simulink model "Guiagem_Cessna_2024_Hinf_MC_2.sil1-89925"  (R2020b)
settings: Solver=FixedStepAuto  StartTime=0.0  StopTime=100  RelTol=1e-3  EnableMultiTasking=on
undefined symbols (not defined in the file): f, K, Kext
libraries: slrealtimeutilitieslib x4, dspnetwork x1, instrumentlib x1, dspswit3 x1
settings Model: Creator=Sergio  LastModifiedBy=amarc
settings SolverCC: ZeroCrossAlgorithm=Non-adaptive  AutoInsertRateTranBlk=on
settings DataIOCC: SaveFormat=Array  SignalLoggingSaveFormat=ModelDataLogs  ReturnWorkspaceOutputs=off
settings OptimizationCC: ExpressionDepthLimit=2147483647  InitFltsAndDblsToZero=on  LifeSpan=inf
settings DebuggingCC: UnderspecifiedInitializationDetection=Classic  MergeDetectMultiDrivingBlocksExec=none  SolverPrmCheckMsg=warning  FcnCallInpInsideContextMsg=warning  StateNameClashWarn=warning  SFUnexpectedBacktrackingDiag=warning  SFNoUnconditionalDefaultTransitionDiag=warning  SFExecutionAtInitializationDiag=none  ArithmeticOperatorsInVariantConditions=warning
settings HardwareCC: ProdBitPerPointer=32  ProdBitPerSizeT=32  ProdBitPerPtrDiffT=32  ProdLargestAtomicFloat=None  ProdIntDivRoundTo=Undefined  ProdEndianess=Unspecified  ProdWordSize=32  ProdHWDeviceType=32-bit Generic
settings ModelReferenceCC: PropagateSignalLabelsOutOfModel=off
settings CodeAppCC: StateflowObjectComments=on
settings GRTTargetCC: TargetLangStandard=C89/C90 (ANSI)  CombineOutputUpdateFcns=off  GRTInterface=on
settings ConfigComp: CovMetricSettings=dw  CovSaveCumulativeToWorkspaceVar=on  CovSaveSingleToWorkspaceVar=on

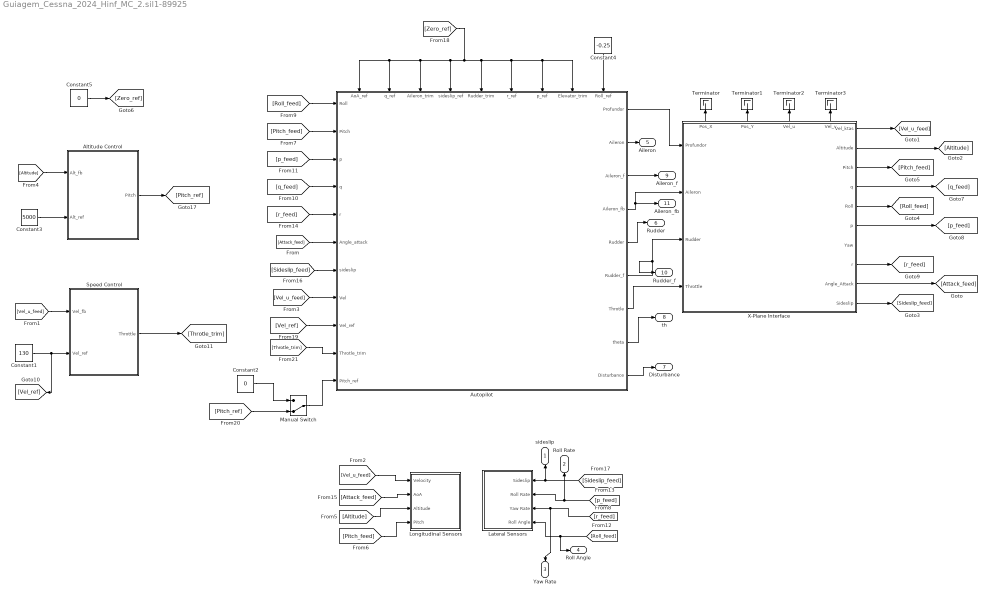
== system Guiagem_Cessna_2024_Hinf_MC_2.sil1-89925 ==
  " X-Plane Interface" : Subsystem
      settings: PortSchema="{\"entries\":[{\"content\":{\"sides\":[{\"content\":{\"connectorIds\":[\"Out11\",\"Out12\",\"Out13\",\"Out14\"]},\"type\":\"ConnectorPlacement.EquallySpacedRectSide\",\"uuid\":\"b287e413-66a9-459c-a605-f8faf73f9bc2\"},{\"content\":{\"connectorIds\":[],\"side\":\"RIGHT\"},\"type\":\"ConnectorPlacement.EquallySpacedRectSide\",\"uuid\":\"a5e9f4a4-94bd-4eea-a928-8343143dc0b5\"},{\"content\":{\"connectorIds\":[\"In1\",\"In2\",\"In3\",\"In4\"],\"side\":\"TOP\"},\"type\":\"ConnectorPlacement.EquallySpacedRectSide\",\"uuid\":\"65fac83d-8715-4b62-9066-f37b198650c3\"},{\"content\":{\"connectorIds\":[\"Out1\",\"Out2\",\"Out3\",\"Out4\",\"Out5\",\"Out6\",\"Out7\",\"Out8\",\"Out9\",\"Out10\"],\"side\":\"BOTTOM\"},\"type\":\"ConnectorPlacement.EquallySpacedRectSide\",\"uuid\":\"a2dcd193-bd07-4351-bec8-c331219c4654\"},{\"content\":{\"connectorIds\":[],\"side\":\"HIDDEN\"},\"type\":\"ConnectorPlacement.EquallySpacedRectSide\",\"uuid\":\"1a5040b2-fe36-41dc-86fb-013b5c75b469\"}]},\"type\":\"ConnectorPlacement.EquallySpacedConnector\",\"uuid\":\"106c77f0-a37d-45d1-adde-f758d3a1985d\"}],\"packageUris\":[\"http://schema.mathworks.com/mf0/Connector/R2020b\"],\"version\":\"1.0\"}"
  Altitude Control : Subsystem
  Autopilot : Subsystem
      settings: PortSchema="{\"entries\":[{\"content\":{\"sides\":[{\"content\":{\"connectorIds\":[\"In1\",\"In2\",\"In3\",\"In4\",\"In5\",\"In6\",\"In7\",\"In8\",\"In9\"]},\"type\":\"ConnectorPlacement.EquallySpacedRectSide\",\"uuid\":\"90d188e5-ac80-4fa1-9be5-1977b7afda35\"},{\"content\":{\"connectorIds\":[],\"side\":\"RIGHT\"},\"type\":\"ConnectorPlacement.EquallySpacedRectSide\",\"uuid\":\"3c236712-b96b-412a-bd89-43ab7dbf8775\"},{\"content\":{\"connectorIds\":[\"In10\",\"In11\",\"In12\",\"In13\",\"In14\",\"In15\",\"In16\",\"In17\",\"In18\",\"In19\",\"In20\"],\"side\":\"TOP\"},\"type\":\"ConnectorPlacement.EquallySpacedRectSide\",\"uuid\":\"6007b185-c294-4b33-95b4-cce134aab69e\"},{\"content\":{\"connectorIds\":[\"Out1\",\"Out2\",\"Out3\",\"Out4\",\"Out5\",\"Out6\",\"Out7\",\"Out8\",\"Out9\"],\"side\":\"BOTTOM\"},\"type\":\"ConnectorPlacement.EquallySpacedRectSide\",\"uuid\":\"8021ee20-ed9f-44e6-9633-5f26e44b493a\"},{\"content\":{\"connectorIds\":[],\"side\":\"HIDDEN\"},\"type\":\"ConnectorPlacement.EquallySpacedRectSide\",\"uuid\":\"d76e2603-a0b8-4e8e-9a67-23be50d7a88d\"}]},\"type\":\"ConnectorPlacement.EquallySpacedConnector\",\"uuid\":\"5cc68935-0bb4-4dc0-b853-f412eb7ddb59\"}],\"packageUris\":[\"http://schema.mathworks.com/mf0/Connector/R2020b\"],\"version\":\"1.0\"}"
  Constant1 : Constant  Value=130
  Constant2 : Constant  Value=0
  Constant3 : Constant  Value=5000
  Constant4 : Constant  Value=-0.25
  Constant5 : Constant  Value=0
  Lateral Sensors : Subsystem
      settings: PortSchema="{\"entries\":[{\"content\":{\"sides\":[{\"content\":{\"connectorIds\":[]},\"type\":\"ConnectorPlacement.EquallySpacedRectSide\",\"uuid\":\"986c3f4b-ed7a-4ad8-bd03-91912b97fe30\"},{\"content\":{\"connectorIds\":[\"In1\",\"In2\",\"In3\",\"In4\"],\"side\":\"RIGHT\"},\"type\":\"ConnectorPlacement.EquallySpacedRectSide\",\"uuid\":\"64bd5685-5cfd-4001-81bc-54a3daf5c9ef\"},{\"content\":{\"connectorIds\":[],\"side\":\"TOP\"},\"type\":\"ConnectorPlacement.EquallySpacedRectSide\",\"uuid\":\"1795adf4-0013-4b9c-8eea-2acf118ad1a4\"},{\"content\":{\"connectorIds\":[],\"side\":\"HIDDEN\"},\"type\":\"ConnectorPlacement.EquallySpacedRectSide\",\"uuid\":\"52ac3bc6-5824-4ddb-b53d-3df0f347e745\"}]},\"type\":\"ConnectorPlacement.EquallySpacedConnector\",\"uuid\":\"dda1921c-f3e4-455c-9a4a-8ad91fc2a8d4\"}],\"packageUris\":[\"http://schema.mathworks.com/mf0/Connector/R2020b\"],\"version\":\"1.0\"}"
  Longitudinal Sensors : Subsystem
  Manual Switch : ManualSwitch  CurrentSetting=0
  Speed Control : Subsystem
  Terminator{,1..3} (4 alike) : Terminator
  sideslip : Outport
  Roll Rate : Outport  Port=2
  Yaw Rate : Outport  Port=3
  Roll Angle : Outport  Port=4
  Aileron : Outport  Port=5
  Rudder : Outport  Port=6
  Disturbance : Outport  Port=7
  th : Outport  Port=8
  Aileron_f : Outport  Port=9
  Rudder_f : Outport  Port=10
  Aileron_fb : Outport  Port=11
  wires:
  Constant1/1 -> Speed Control/1(Vel_ref), [Vel_ref]
  Constant3/1 -> Altitude Control/2(Alt_ref)
  " X-Plane Interface"/9(Angle_Attack) -> [Attack_feed]
  [Attack_feed] -> Autopilot/15(Angle_attack)
  " X-Plane Interface"/1(Vel_ktas) -> [Vel_u_feed]
  [Vel_u_feed] -> Longitudinal Sensors/1(Velocity)
  [Vel_u_feed] -> Autopilot/17(Vel)
  " X-Plane Interface"/2(Altitude) -> [Altitude]
  [Altitude] -> Altitude Control/1(Alt_fb)
  [Altitude] -> Longitudinal Sensors/3(Altitude)
  " X-Plane Interface"/3(Pitch) -> [Pitch_feed]
  [Pitch_feed] -> Longitudinal Sensors/4(Pitch)
  [Pitch_feed] -> Autopilot/11(Pitch)
  " X-Plane Interface"/4(q) -> [q_feed]
  [q_feed] -> Autopilot/13(q)
  " X-Plane Interface"/5(Roll) -> [Roll_feed]
  [Roll_feed] -> Autopilot/10(Roll)
  [Roll_feed] -> Roll Angle/1, Lateral Sensors/4(Roll Angle)
  " X-Plane Interface"/6(p) -> [p_feed]
  [p_feed] -> Autopilot/12(p)
  " X-Plane Interface"/8(r) -> [r_feed]
  [r_feed] -> Autopilot/14(r)
  [Attack_feed] -> Longitudinal Sensors/2(AoA)
  " X-Plane Interface"/10(Sideslip) -> [Sideslip_feed]
  [Sideslip_feed] -> Autopilot/16(sideslip)
  Autopilot/1(Profundor) -> " X-Plane Interface"/1(Profundor)
  Autopilot/4(Aileron_fb) -> " X-Plane Interface"/2(Aileron), Aileron_fb/1
  Autopilot/6(Rudder_f) -> Rudder_f/1, " X-Plane Interface"/3(Rudder)
  Autopilot/7(Throtle) -> " X-Plane Interface"/4(Throttle)
  [Sideslip_feed] -> sideslip/1, Lateral Sensors/1(Sideslip)
  [p_feed] -> Roll Rate/1, Lateral Sensors/2(Roll Rate)
  [r_feed] -> Yaw Rate/1, Lateral Sensors/3(Yaw Rate)
  Manual Switch/1 -> Autopilot/20(Pitch_ref)
  Constant2/1 -> Manual Switch/1
  [Pitch_ref] -> Manual Switch/2
  Altitude Control/1(Pitch) -> [Pitch_ref]
  Constant5/1 -> [Zero_ref]
  [Vel_ref] -> Autopilot/18(Vel_ref)
  [Zero_ref] -> Autopilot/8(Elevator_trim), Autopilot/7(p_ref), Autopilot/6(r_ref), Autopilot/5(Rudder_trim), Autopilot/4(sideslip_ref), Autopilot/3(Aileron_trim), Autopilot/2(q_ref), Autopilot/1(AoA_ref)
  " X-Plane Interface"/11(Pos_X) -> Terminator/1
  " X-Plane Interface"/12(Pos_Y) -> Terminator1/1
  " X-Plane Interface"/13(Vel_u) -> Terminator2/1
  " X-Plane Interface"/14(Vel_v) -> Terminator3/1
  [Throtle_trim] -> Autopilot/19(Throtle_trim)
  Speed Control/1(Throttle) -> [Throtle_trim]
  [Vel_u_feed] -> Speed Control/2(Vel_fb)
  Autopilot/9(Disturbance) -> Disturbance/1
  Autopilot/8(theta) -> th/1
  Constant4/1 -> Autopilot/9(Roll_ref)
  Autopilot/2(Aileron) -> Aileron/1
  Autopilot/5(Rudder) -> Rudder/1
  Autopilot/3(Aileron_f) -> Aileron_f/1

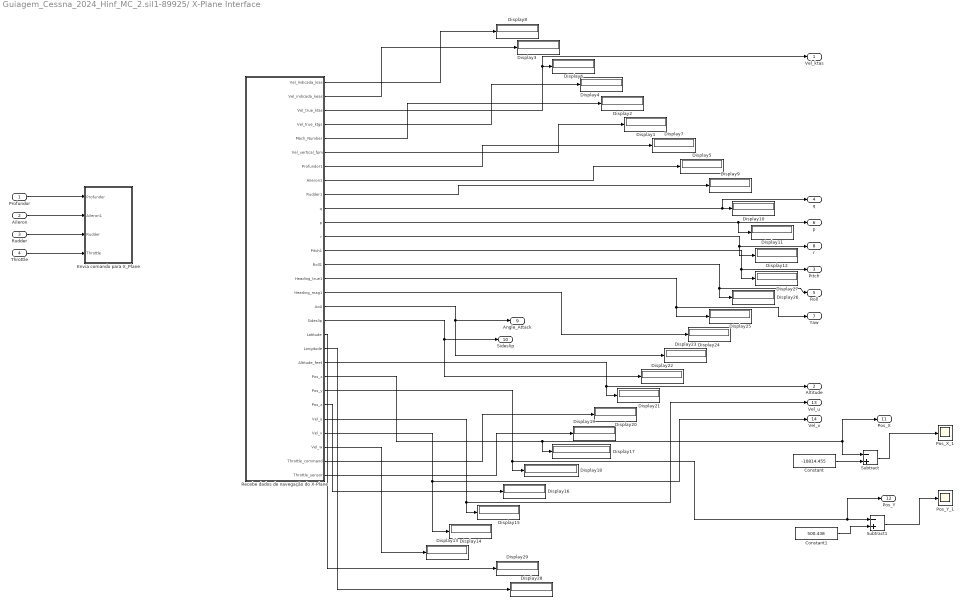
== system Guiagem_Cessna_2024_Hinf_MC_2.sil1-89925/ X-Plane Interface ==
  Profundor : Inport
  Aileron : Inport  Port=2
  Rudder : Inport  Port=3
  Throttle : Inport  Port=4
  Constant : Constant  Value=-10814.455
  Constant1 : Constant  Value=500.438
  Display{1..29} (29 alike) : Display
  Envia comando para X_Plane : Subsystem
  Pos_X_1 : Scope
  Pos_Y_1 : Scope
  Recebe dados de navegação do X-Plane : Subsystem
  Subtract : Sum  Inputs=-+
  Subtract1 : Sum  Inputs=-+
  Vel_ktas : Outport
  Altitude : Outport  Port=2
  Pitch : Outport  Port=3
  q : Outport  Port=4
  Roll : Outport  Port=5
  p : Outport  Port=6
  Yaw : Outport  Port=7
  r : Outport  Port=8
  Angle_Attack : Outport  Port=9
  Sideslip : Outport  Port=10
  Pos_X : Outport  Port=11
  Pos_Y : Outport  Port=12
  Vel_u : Outport  Port=13
  Vel_v : Outport  Port=14
  wires:
  Recebe dados de navegação do X-Plane/13(Pitch1) -> Display27/1, Pitch/1
  Recebe dados de navegação do X-Plane/16(Heading_mag1) -> Display24/1
  Recebe dados de navegação do X-Plane/15(Heading_true1) -> Display25/1, Yaw/1
  Recebe dados de navegação do X-Plane/21(Altitude_feet) -> Display21/1, Altitude/1
  Recebe dados de navegação do X-Plane/12(r) -> Display12/1, r/1
  Recebe dados de navegação do X-Plane/9(Rudder1) -> Display9/1
  Recebe dados de navegação do X-Plane/25(Vel_u) -> Display15/1, Vel_u/1
  Recebe dados de navegação do X-Plane/17(AoA) -> Angle_Attack/1, Display23/1
  Recebe dados de navegação do X-Plane/10(q) -> q/1, Display10/1
  Recebe dados de navegação do X-Plane/22(Pos_x) -> Display17/1, Subtract/1, Pos_X/1
  Recebe dados de navegação do X-Plane/18(Sideslip) -> Sideslip/1, Display22/1
  Recebe dados de navegação do X-Plane/1(Vel_Indicada_kias) -> Display8/1
  Recebe dados de navegação do X-Plane/29(Throttle_sensor) -> Display19/1
  Recebe dados de navegação do X-Plane/24(Pos_z) -> Display16/1
  Recebe dados de navegação do X-Plane/14(Roll1) -> Display26/1, Roll/1
  Recebe dados de navegação do X-Plane/28(Throttle_command) -> Display20/1
  Recebe dados de navegação do X-Plane/27(Vel_w) -> Display13/1
  Recebe dados de navegação do X-Plane/23(Pos_y) -> Display18/1, Pos_Y/1, Subtract1/1
  Recebe dados de navegação do X-Plane/11(p) -> Display11/1, p/1
  Recebe dados de navegação do X-Plane/6(Vel_vertical_fpm) -> Display1/1
  Recebe dados de navegação do X-Plane/2(Vel_indicada_keas) -> Display3/1
  Recebe dados de navegação do X-Plane/8(Aileron1) -> Display5/1
  Recebe dados de navegação do X-Plane/4(Vel_true_ktgs) -> Display4/1
  Recebe dados de navegação do X-Plane/3(Vel_true_ktas) -> Vel_ktas/1, Display6/1
  Recebe dados de navegação do X-Plane/26(Vel_v) -> Display14/1, Vel_v/1
  Recebe dados de navegação do X-Plane/5(Mach_Number) -> Display2/1
  Recebe dados de navegação do X-Plane/7(Profundor1) -> Display7/1
  Subtract/1 -> Pos_X_1/1
  Constant/1 -> Subtract/2
  Constant1/1 -> Subtract1/2
  Subtract1/1 -> Pos_Y_1/1
  Recebe dados de navegação do X-Plane/19(Latitude) -> Display29/1
  Recebe dados de navegação do X-Plane/20(Longitude) -> Display28/1
  Profundor/1 -> Envia comando para X_Plane/1(Profundor)
  Aileron/1 -> Envia comando para X_Plane/2(Aileron1)
  Rudder/1 -> Envia comando para X_Plane/3(Rudder)
  Throttle/1 -> Envia comando para X_Plane/4(Throttle)

== system Guiagem_Cessna_2024_Hinf_MC_2.sil1-89925/Altitude Control ==
  Alt_fb : Inport
  Alt_ref : Inport  Port=2
  Display : Display
  Gain : Gain
  PID Altitude : Subsystem
  Sum2 : Sum  Inputs=|+-  SaturateOnIntegerOverflow=on
  Pitch : Outport
  wires:
  PID Altitude/1(ea) -> Gain/1
  Sum2/1 -> Display/1, PID Altitude/1(e_theta)
  Alt_ref/1 -> Sum2/1
  Alt_fb/1 -> Sum2/2
  Gain/1 -> Pitch/1

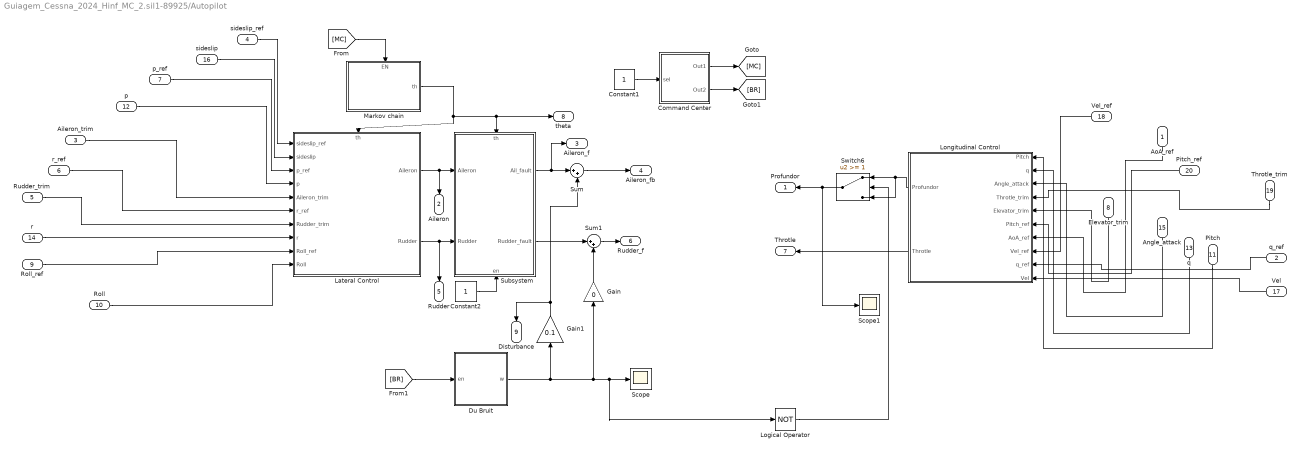
== system Guiagem_Cessna_2024_Hinf_MC_2.sil1-89925/Autopilot ==
  AoA_ref : Inport
  q_ref : Inport  Port=2
  Aileron_trim : Inport  Port=3
  sideslip_ref : Inport  Port=4
  Rudder_trim : Inport  Port=5
  r_ref : Inport  Port=6
  p_ref : Inport  Port=7
  Elevator_trim : Inport  Port=8
  Roll_ref : Inport  Port=9
  Roll : Inport  Port=10
  Pitch : Inport  Port=11
  p : Inport  Port=12
  q : Inport  Port=13
  r : Inport  Port=14
  Angle_attack : Inport  Port=15
  sideslip : Inport  Port=16
  Vel : Inport  Port=17
  Vel_ref : Inport  Port=18
  Throtle_trim : Inport  Port=19
  Pitch_ref : Inport  Port=20
  Command Center : Subsystem
  Constant1 : Constant
  Constant2 : Constant
  Du Bruit : Subsystem
  Gain : Gain  Gain=0
  Gain1 : Gain  Gain=0.1
  Lateral Control : Subsystem
      settings: PortSchema="{\"entries\":[{\"content\":{\"sides\":[{\"content\":{\"connectorIds\":[\"In1\",\"In2\",\"In3\",\"In4\",\"In5\",\"In6\",\"In7\",\"In8\",\"In9\",\"In10\"]},\"type\":\"ConnectorPlacement.EquallySpacedRectSide\",\"uuid\":\"81480b8d-acf9-4486-b64d-17d5a3a359c2\"},{\"content\":{\"connectorIds\":[\"Out1\",\"Out2\"],\"side\":\"RIGHT\"},\"type\":\"ConnectorPlacement.EquallySpacedRectSide\",\"uuid\":\"f51d7c70-ae43-4c04-b132-323ecb9750c2\"},{\"content\":{\"connectorIds\":[\"In11\"],\"side\":\"TOP\"},\"type\":\"ConnectorPlacement.EquallySpacedRectSide\",\"uuid\":\"e45e99c5-9997-4ec4-be29-da73ef44331d\"},{\"content\":{\"connectorIds\":[],\"side\":\"HIDDEN\"},\"type\":\"ConnectorPlacement.EquallySpacedRectSide\",\"uuid\":\"472f75da-d9b5-4c89-82f1-bd7b45161ec6\"}]},\"type\":\"ConnectorPlacement.EquallySpacedConnector\",\"uuid\":\"4f90d613-2ea4-447f-9646-109b9180330b\"}],\"packageUris\":[\"http://schema.mathworks.com/mf0/Connector/R2020b\"],\"version\":\"1.0\"}"
  Logical Operator : Logic  Operator=NOT  AllPortsSameDT=off  OutDataTypeStr=boolean
  Longitudinal Control : Subsystem
  Markov chain : Subsystem
      settings: PortSchema="{\"entries\":[{\"content\":{\"sides\":[{\"content\":{\"connectorIds\":[]},\"type\":\"ConnectorPlacement.EquallySpacedRectSide\",\"uuid\":\"80710c7a-07e6-43ae-a398-972a0eb5af13\"},{\"content\":{\"connectorIds\":[\"Out1\"],\"side\":\"RIGHT\"},\"type\":\"ConnectorPlacement.EquallySpacedRectSide\",\"uuid\":\"28b5b092-7e5d-428e-90bd-fdf9ff161332\"},{\"content\":{\"connectorIds\":[\"In1\"],\"side\":\"TOP\"},\"type\":\"ConnectorPlacement.EquallySpacedRectSide\",\"uuid\":\"22863cb7-627c-45e7-8d90-71727f39a809\"},{\"content\":{\"connectorIds\":[],\"side\":\"HIDDEN\"},\"type\":\"ConnectorPlacement.EquallySpacedRectSide\",\"uuid\":\"e7671043-5e22-4c27-8279-fe6d843a7844\"}]},\"type\":\"ConnectorPlacement.EquallySpacedConnector\",\"uuid\":\"bc28ef5d-b311-4d28-80fd-097e2dffd910\"}],\"packageUris\":[\"http://schema.mathworks.com/mf0/Connector/R2020b\"],\"version\":\"1.0\"}"
  Scope : Scope
  Scope1 : Scope
  Subsystem : Subsystem
      settings: PortSchema="{\"entries\":[{\"content\":{\"sides\":[{\"content\":{\"connectorIds\":[\"In1\",\"In2\"]},\"type\":\"ConnectorPlacement.EquallySpacedRectSide\",\"uuid\":\"51a358d2-0277-4e02-9bc5-d86ec75e586a\"},{\"content\":{\"connectorIds\":[\"Out1\",\"Out2\"],\"side\":\"RIGHT\"},\"type\":\"ConnectorPlacement.EquallySpacedRectSide\",\"uuid\":\"48fac5f6-d3f7-4a23-9035-dace107cd9ad\"},{\"content\":{\"connectorIds\":[\"In3\"],\"side\":\"TOP\"},\"type\":\"ConnectorPlacement.EquallySpacedRectSide\",\"uuid\":\"fe2b725a-5173-4175-81cd-54f0c8666ca6\"},{\"content\":{\"connectorIds\":[\"In4\"],\"side\":\"BOTTOM\"},\"type\":\"ConnectorPlacement.EquallySpacedRectSide\",\"uuid\":\"7335eb3f-eaf6-4179-b795-6b8ea5857190\"},{\"content\":{\"connectorIds\":[],\"side\":\"HIDDEN\"},\"type\":\"ConnectorPlacement.EquallySpacedRectSide\",\"uuid\":\"2585f13a-08e3-4863-882a-f65ebe29ac28\"}]},\"type\":\"ConnectorPlacement.EquallySpacedConnector\",\"uuid\":\"792a0ec4-d064-45f9-9106-30d8e1278945\"}],\"packageUris\":[\"http://schema.mathworks.com/mf0/Connector/R2020b\"],\"version\":\"1.0\"}"
  Sum : Sum  Inputs=|++
  Sum1 : Sum  Inputs=|++
  Switch6 : Switch  Threshold=1
  Profundor : Outport
  Aileron : Outport  Port=2
  Aileron_f : Outport  Port=3
  Aileron_fb : Outport  Port=4
  Rudder : Outport  Port=5
  Rudder_f : Outport  Port=6
  Throtle : Outport  Port=7
  theta : Outport  Port=8
  Disturbance : Outport  Port=9
  wires:
  Pitch/1 -> Longitudinal Control/1(Pitch)
  q/1 -> Longitudinal Control/2(q)
  Angle_attack/1 -> Longitudinal Control/3(Angle_attack)
  Throtle_trim/1 -> Longitudinal Control/4(Throtle_trim)
  Elevator_trim/1 -> Longitudinal Control/5(Elevator_trim)
  Pitch_ref/1 -> Longitudinal Control/6(Pitch_ref)
  AoA_ref/1 -> Longitudinal Control/7(AoA_ref)
  Vel_ref/1 -> Longitudinal Control/8(Vel_ref)
  q_ref/1 -> Longitudinal Control/9(q_ref)
  Vel/1 -> Longitudinal Control/10(Vel)
  sideslip_ref/1 -> Lateral Control/1(sideslip_ref)
  sideslip/1 -> Lateral Control/2(sideslip)
  p_ref/1 -> Lateral Control/3(p_ref)
  p/1 -> Lateral Control/4(p)
  Aileron_trim/1 -> Lateral Control/5(Aileron_trim)
  r_ref/1 -> Lateral Control/6(r_ref)
  Rudder_trim/1 -> Lateral Control/7(Rudder_trim)
  r/1 -> Lateral Control/8(r)
  Roll_ref/1 -> Lateral Control/9(Roll_ref)
  Roll/1 -> Lateral Control/10(Roll)
  Lateral Control/1(Aileron) -> Subsystem/1(Aileron), Aileron/1
  Longitudinal Control/2(Throtle) -> Throtle/1
  Lateral Control/2(Rudder) -> Rudder/1, Subsystem/2(Rudder)
  Subsystem/1(Ail_fault) -> Aileron_f/1, Sum/1
  Sum/1 -> Aileron_fb/1
  Subsystem/2(Rudder_fault) -> Sum1/1
  Gain/1 -> Sum1/2
  [MC] -> Markov chain/1(EN)
  Markov chain/1(th) -> theta/1, Subsystem/3(th), Lateral Control/11(th)
  Constant1/1 -> Command Center/1(sel)
  Command Center/2(Out2) -> [BR]
  Command Center/1(Out1) -> [MC]
  Gain1/1 -> Sum/2, Disturbance/1
  [BR] -> Du Bruit/1(en)
  Constant2/1 -> Subsystem/4(en)
  Sum1/1 -> Rudder_f/1
  Switch6/1 -> Scope1/1, Profundor/1
  Longitudinal Control/1(Profundor) -> Switch6/3, Switch6/1
  Du Bruit/1(w) -> Gain1/1, Gain/1, Logical Operator/1, Scope/1
  Logical Operator/1 -> Switch6/2

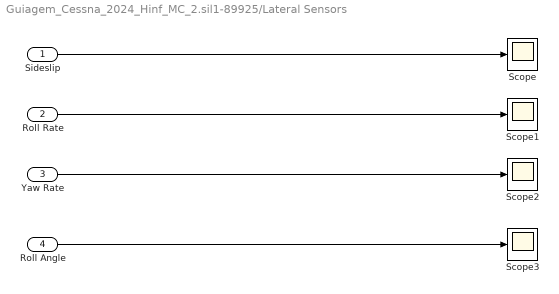
== system Guiagem_Cessna_2024_Hinf_MC_2.sil1-89925/Lateral Sensors ==
  Sideslip : Inport
  Roll Rate : Inport  Port=2
  Yaw Rate : Inport  Port=3
  Roll Angle : Inport  Port=4
  Scope{,1..3} (4 alike) : Scope
  wires:
  Sideslip/1 -> Scope/1
  Roll Rate/1 -> Scope1/1
  Roll Angle/1 -> Scope3/1
  Yaw Rate/1 -> Scope2/1

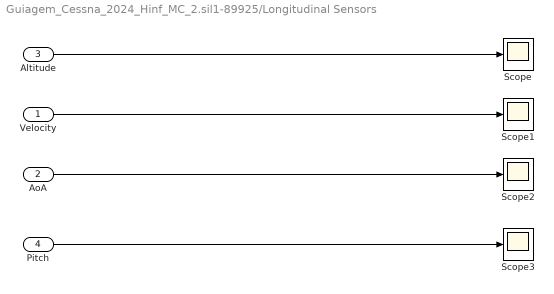
== system Guiagem_Cessna_2024_Hinf_MC_2.sil1-89925/Longitudinal Sensors ==
  Velocity : Inport
  AoA : Inport  Port=2
  Altitude : Inport  Port=3
  Pitch : Inport  Port=4
  Scope{,1..3} (4 alike) : Scope
  wires:
  Altitude/1 -> Scope/1
  Velocity/1 -> Scope1/1
  AoA/1 -> Scope2/1
  Pitch/1 -> Scope3/1

== system Guiagem_Cessna_2024_Hinf_MC_2.sil1-89925/Speed Control ==
  Vel_ref : Inport
  Vel_fb : Inport  Port=2
  PID Velocidade : Subsystem
  Sum7 : Sum  Inputs=|+-
  Throttle : Outport
  wires:
  Vel_fb/1 -> Sum7/2
  PID Velocidade/1(ev) -> Throttle/1
  Vel_ref/1 -> Sum7/1
  Sum7/1 -> PID Velocidade/1(e_vel)

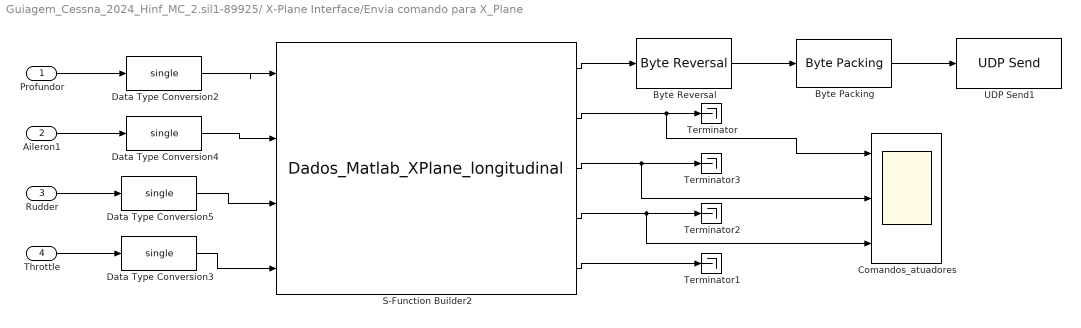
== system Guiagem_Cessna_2024_Hinf_MC_2.sil1-89925/ X-Plane Interface/Envia comando para X_Plane ==
  Profundor : Inport
  Aileron1 : Inport  Port=2
  Rudder : Inport  Port=3
  Throttle : Inport  Port=4
  Byte Packing : slrealtimeutilitieslib/Byte Packing  MaskPackedDataType=uint8  MaskUnpackedDataTypes={'uint8'}  MaskAlignment=1
  Byte Reversal : slrealtimeutilitieslib/Byte Reversal  numInp=1
      settings: SourceProductBaseCode=XP
  Comandos_atuadores : Scope  NumInputPorts=3
  Data Type Conversion{2..5} (4 alike) : DataTypeConversion  OutDataTypeStr=single  SaturateOnIntegerOverflow=on
  S-Function Builder2 : S-Function  InitFcn=try, set_param(gcb,'FunctionName','Dados_Matlab_XPlane_longitudinal'), end  FunctionName=Dados_Matlab_XPlane_longitudinal  SFunctionModules=Dados_Matlab_XPlane_longitudinal_wrapper  SFunctionDeploymentMode=off  EnableBusSupport=off  mask(S-Function Builder){}
      mask help: The S-Function Builder block creates a wrapper C-MEX S-function from your supplied C code with multiple input ports, output ports, and a variable number of scalar, vector, or matrix parameters. The input and output ports can propagate Simulink built-in data types, fixed-point datatypes, complex, frame, 1-D, and 2-D signals. This block also supports discrete and continuous states of type real. You can optionally have the block generate a TLC file to be used with Real-Time Workshop for code generation.
      mask init:
      | val = [[.9  0.75 0.75 1 1 .9 .9 1]',[1 1 0.75 0.75 .9 .9 1 .9]'];try , sys = get_param(gcb,'SfunBuilderFcnName');if isempty(sys), sys = get_param(gcb,'FunctionName'); end,catch, sys = get_param(gcb,'FunctionName'); end
      settings: CopyFcn=set_param(gcbh,'LinkStatus','none')  PreSaveFcn=try, set_param(gcb,'FunctionName','Dados_Matlab_XPlane_longitudinal'), end  OpenFcn=sfunctionwizard(gcbh)
      mask Display: plot(val(:,1),val(:,2)),disp(sys),port_label('input',1,'Profundor'),port_label('input',2,'Aileron'),port_label('input',3,'Rudder'),port_label('input',4,'Throttle'),port_label('output',1,'Atuadores_Out'),port_label('output',2,'elevator_out'),port_label('output',3,'aileron_out'),port_label('output',4,'rudder_out'),port_label('output',5,'throttle_out')
  Terminator{,1..3} (4 alike) : Terminator
  UDP Send1 : dspnetwork/UDP Send  remoteURL='161.24.191.101'  remotePort=49000  localURL='0.0.0.0'  localPortSource=Automatically determine  localPort=-1  sendBufferSize=113  sampletime=-1  blockPlatform=[]  separateLengthPort=0
  wires:
  Data Type Conversion5/1 -> S-Function Builder2/3
  S-Function Builder2/2 -> Terminator/1, Comandos_atuadores/1
  Rudder/1 -> Data Type Conversion5/1
  Aileron1/1 -> Data Type Conversion4/1
  S-Function Builder2/5 -> Terminator1/1
  S-Function Builder2/4 -> Terminator2/1, Comandos_atuadores/3
  S-Function Builder2/3 -> Terminator3/1, Comandos_atuadores/2
  Profundor/1 -> Data Type Conversion2/1
  Byte Reversal/1 -> Byte Packing/1
  Data Type Conversion2/1 -> S-Function Builder2/1
  Data Type Conversion4/1 -> S-Function Builder2/2
  S-Function Builder2/1 -> Byte Reversal/1
  Data Type Conversion3/1 -> S-Function Builder2/4
  Byte Packing/1 -> UDP Send1/1
  Throttle/1 -> Data Type Conversion3/1

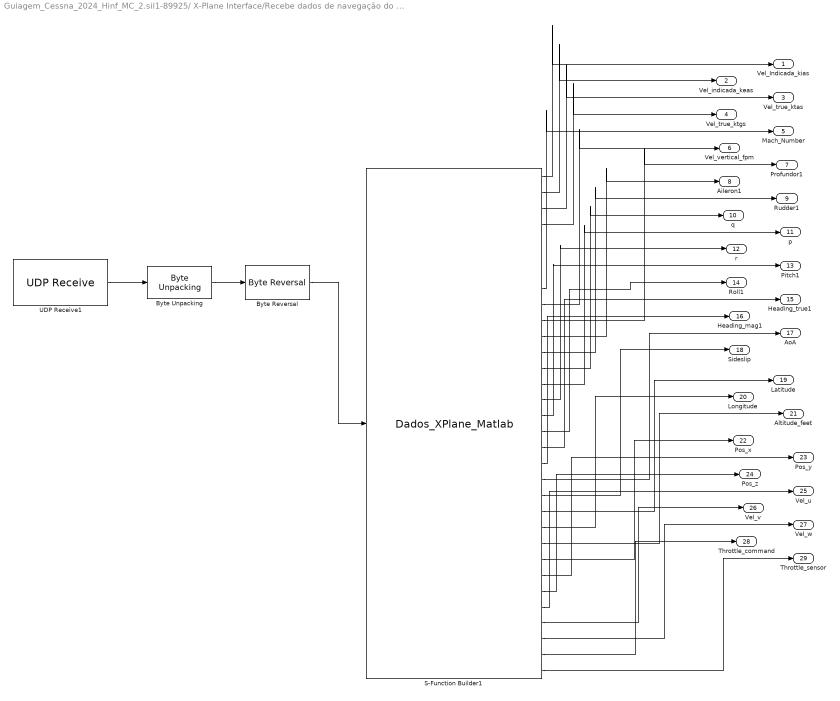
== system Guiagem_Cessna_2024_Hinf_MC_2.sil1-89925/ X-Plane Interface/Recebe dados de navegação do X-Plane ==
  Byte Reversal : slrealtimeutilitieslib/Byte Reversal  numInp=1
      settings: SourceProductBaseCode=XP
  Byte Unpacking : slrealtimeutilitieslib/Byte Unpacking  MaskUnpackedDataTypes={'uint8'}  MaskUnpackedDataSizes={[1, 365]}  MaskAlignment=1
      settings: SourceProductBaseCode=XP
  S-Function Builder1 : S-Function  InitFcn=try, set_param(gcb,'FunctionName','Dados_XPlane_Matlab'), end  FunctionName=Dados_XPlane_Matlab  SFunctionModules=Dados_XPlane_Matlab_wrapper  SFunctionDeploymentMode=off  EnableBusSupport=off  mask(S-Function Builder){}
      mask help: The S-Function Builder block creates a wrapper C-MEX S-function from your supplied C code with multiple input ports, output ports, and a variable number of scalar, vector, or matrix parameters. The input and output ports can propagate Simulink built-in data types, fixed-point datatypes, complex, frame, 1-D, and 2-D signals. This block also supports discrete and continuous states of type real. You can optionally have the block generate a TLC file to be used with Real-Time Workshop for code generation.
      mask init: same as Guiagem_Cessna_2024_Hinf_MC_2.sil1-89925/ X-Plane Interface/Envia comando para X_Plane/S-Function Builder2
      settings: CopyFcn=set_param(gcbh,'LinkStatus','none')  PreSaveFcn=try, set_param(gcb,'FunctionName','Dados_XPlane_Matlab'), end  OpenFcn=sfunctionwizard(gcbh)
      mask Display: plot(val(:,1),val(:,2)),disp(sys),port_label('input',1,'Dados_in'),port_label('output',1,'Vind_kias'),port_label('output',2,'Vind_keas'),port_label('output',3,'Vtrue_ktas'),port_label('output',4,'Vtrue_ktgs'),port_label('output',5,'Vind_mph'),port_label('output',6,'Vtrue_mphas'),port_label('output',7,'Vtrue_mphgs'),port_label('output',8,'Mach'),port_label('output',9,'VVI'),port_label('output',10,'Elevator'),port_label('output',11,'Aileron'),port_label('output',12,'Rudder'),port_label('output',13,'Q'),port_label('output',14,'P'),port_label('output',15,'R'),port_label('output',16,'Pitch'),port_label('output',17,'Roll'),port_label('output',18,'Heading_true'),port_label('output',19,'Heading_mag'),port_label('output',20,'AoA'),port_label('output',21,'Sideslip'),port_label('output',22,'Latitude'),port_label('output',23,'Longitude'),port_label('output',24,'Altitude'),port_label('output',25,'X'),port_label('output',26,'Y'),port_label('output',27,'Z'),port_label('output',28,'Vu'),port_label('output',29,'Vv'),port_label('output',30,'Vw'),port_label('output',31,'Throtle_com'),port_label('output',32,'Throtle_sen')
  UDP Receive1 : instrumentlib/UDP Receive  Host=161.24.191.101  Port=49001  LocalPort=49001  EnablePortSharing=off  GetLatestData=off  DataSize=365  DataType=uint8  ASCIIFormatting=%f,  Terminator=LF  ByteOrder=BigEndian  EnableBlockingMode=on  Timeout=5  SampleTime=0.01  LocalAddress=161.24.191.100
  Vel_Indicada_kias : Outport
  Vel_indicada_keas : Outport  Port=2
  Vel_true_ktas : Outport  Port=3
  Vel_true_ktgs : Outport  Port=4
  Mach_Number : Outport  Port=5
  Vel_vertical_fpm : Outport  Port=6
  Profundor1 : Outport  Port=7
  Aileron1 : Outport  Port=8
  Rudder1 : Outport  Port=9
  q : Outport  Port=10
  p : Outport  Port=11
  r : Outport  Port=12
  Pitch1 : Outport  Port=13
  Roll1 : Outport  Port=14
  Heading_true1 : Outport  Port=15
  Heading_mag1 : Outport  Port=16
  AoA : Outport  Port=17
  Sideslip : Outport  Port=18
  Latitude : Outport  Port=19
  Longitude : Outport  Port=20
  Altitude_feet : Outport  Port=21
  Pos_x : Outport  Port=22
  Pos_y : Outport  Port=23
  Pos_z : Outport  Port=24
  Vel_u : Outport  Port=25
  Vel_v : Outport  Port=26
  Vel_w : Outport  Port=27
  Throttle_command : Outport  Port=28
  Throttle_sensor : Outport  Port=29
  wires:
  Byte Unpacking/1 -> Byte Reversal/1
  Byte Reversal/1 -> S-Function Builder1/1
  UDP Receive1/1 -> Byte Unpacking/1
  S-Function Builder1/1 -> Vel_Indicada_kias/1
  S-Function Builder1/2 -> Vel_indicada_keas/1
  S-Function Builder1/3 -> Vel_true_ktas/1
  S-Function Builder1/4 -> Vel_true_ktgs/1
  S-Function Builder1/10 -> Profundor1/1
  S-Function Builder1/8 -> Mach_Number/1
  S-Function Builder1/9 -> Vel_vertical_fpm/1
  S-Function Builder1/11 -> Aileron1/1
  S-Function Builder1/12 -> Rudder1/1
  S-Function Builder1/13 -> q/1
  S-Function Builder1/14 -> p/1
  S-Function Builder1/15 -> r/1
  S-Function Builder1/16 -> Pitch1/1
  S-Function Builder1/17 -> Roll1/1
  S-Function Builder1/18 -> Heading_true1/1
  S-Function Builder1/19 -> Heading_mag1/1
  S-Function Builder1/20 -> AoA/1
  S-Function Builder1/21 -> Sideslip/1
  S-Function Builder1/22 -> Latitude/1
  S-Function Builder1/23 -> Longitude/1
  S-Function Builder1/24 -> Altitude_feet/1
  S-Function Builder1/25 -> Pos_x/1
  S-Function Builder1/26 -> Pos_y/1
  S-Function Builder1/27 -> Pos_z/1
  S-Function Builder1/28 -> Vel_u/1
  S-Function Builder1/29 -> Vel_v/1
  S-Function Builder1/30 -> Vel_w/1
  S-Function Builder1/31 -> Throttle_command/1
  S-Function Builder1/32 -> Throttle_sensor/1

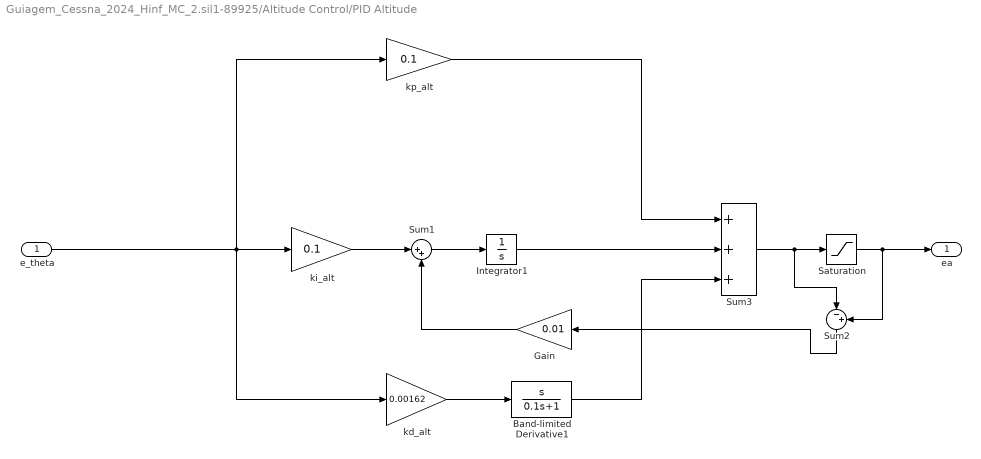
== system Guiagem_Cessna_2024_Hinf_MC_2.sil1-89925/Altitude Control/PID Altitude ==
  e_theta : Inport
  Band-limited Derivative1 : TransferFcn  Numerator=[1 0]  Denominator=[0.1 1]
  Gain : Gain  Gain=0.01
  Integrator1 : Integrator
  Saturation : Saturate  UpperLimit=800  LowerLimit=-800
  Sum1 : Sum  Inputs=|++
  Sum2 : Sum  Inputs=|-+
  Sum3 : Sum  Inputs=+++  InputSameDT=on  SaturateOnIntegerOverflow=on  OutDataTypeStr=Inherit: Same as first input
  kd_alt : Gain  Gain=0.00162  SaturateOnIntegerOverflow=on  OutDataTypeStr=Inherit: Same as input  ParamDataTypeStr=Inherit: Same as input
  ki_alt : Gain  Gain=0.1  SaturateOnIntegerOverflow=on  OutDataTypeStr=Inherit: Same as input  ParamDataTypeStr=Inherit: Same as input
  kp_alt : Gain  Gain=0.1  SaturateOnIntegerOverflow=on  OutDataTypeStr=Inherit: Same as input  ParamDataTypeStr=Inherit: Same as input
  ea : Outport
  wires:
  kp_alt/1 -> Sum3/1
  Band-limited Derivative1/1 -> Sum3/3
  e_theta/1 -> ki_alt/1, kd_alt/1, kp_alt/1
  kd_alt/1 -> Band-limited Derivative1/1
  Integrator1/1 -> Sum3/2
  Sum3/1 -> Sum2/1, Saturation/1
  Saturation/1 -> Sum2/2, ea/1
  ki_alt/1 -> Sum1/1
  Sum1/1 -> Integrator1/1
  Sum2/1 -> Gain/1
  Gain/1 -> Sum1/2

== system Guiagem_Cessna_2024_Hinf_MC_2.sil1-89925/Autopilot/Command Center ==
  sel : Inport
  Demux : Demux  Outputs=2
  MATLAB Function : MATLAB Function  TreatAsAtomicUnit=on
  Out1 : Outport
  Out2 : Outport  Port=2
  wires:
  MATLAB Function/1(y) -> Demux/1
  Demux/1 -> Out1/1
  sel/1 -> MATLAB Function/1(sel)
  Demux/2 -> Out2/1

== system Guiagem_Cessna_2024_Hinf_MC_2.sil1-89925/Autopilot/Du Bruit ==
  en : Inport
  Counter : dspswit3/Counter  Direction=Up  CountEvent=Non-zero sample  CounterSize=User defined  MaxCount=301  InitialCount=0  Output=Count and Hit  HitValue=32  ResetInput=off  SamplesPerFrame=1  Ts=1  CntDtype=double  HitDtype=Logical
  Delay : Delay  DelayLength=1
  MATLAB Function : MATLAB Function  TreatAsAtomicUnit=on
  w : Outport
  wires:
  MATLAB Function/1(w) -> w/1, Delay/1
  Counter/1 -> MATLAB Function/2(cnt)
  Delay/1 -> Counter/1
  en/1 -> MATLAB Function/1(en)

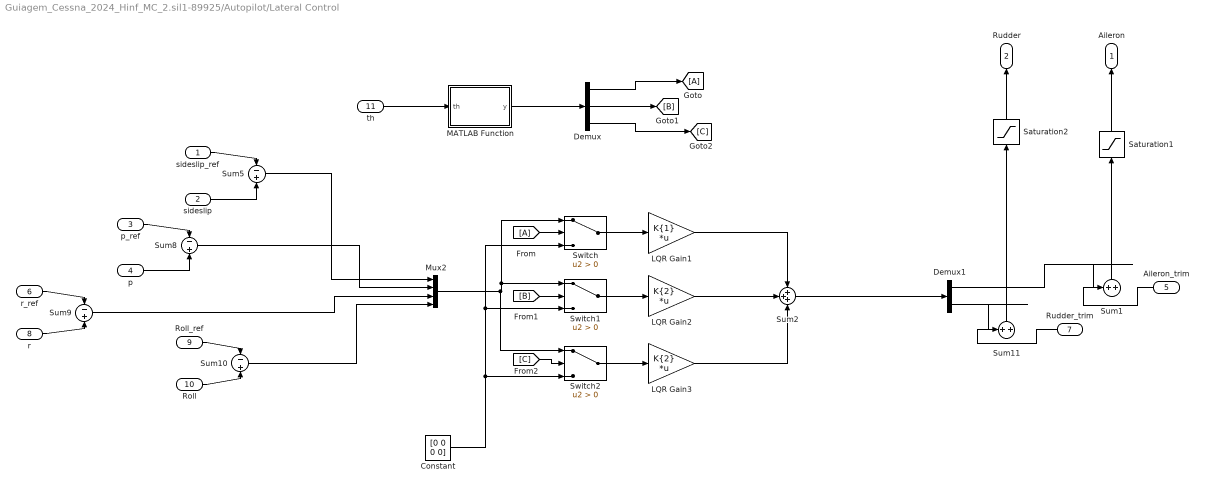
== system Guiagem_Cessna_2024_Hinf_MC_2.sil1-89925/Autopilot/Lateral Control ==
  sideslip_ref : Inport
  sideslip : Inport  Port=2
  p_ref : Inport  Port=3
  p : Inport  Port=4
  Aileron_trim : Inport  Port=5
  r_ref : Inport  Port=6
  Rudder_trim : Inport  Port=7
  r : Inport  Port=8
  Roll_ref : Inport  Port=9
  Roll : Inport  Port=10
  th : Inport  Port=11
  Constant : Constant  Value=[0 0 0 0]  VectorParams1D=off
  Demux : Demux  Outputs=3
  Demux1 : Demux  Outputs=2
  LQR Gain1 : Gain  Gain=K{1}  Multiplication=Matrix(K*u) (u vector)  SaturateOnIntegerOverflow=on  OutDataTypeStr=Inherit: Same as input  ParamDataTypeStr=Inherit: Same as input
  LQR Gain2 : Gain  Gain=K{2}  Multiplication=Matrix(K*u) (u vector)  SaturateOnIntegerOverflow=on  OutDataTypeStr=Inherit: Same as input  ParamDataTypeStr=Inherit: Same as input
  LQR Gain3 : Gain  Gain=K{2}  Multiplication=Matrix(K*u) (u vector)  SaturateOnIntegerOverflow=on  OutDataTypeStr=Inherit: Same as input  ParamDataTypeStr=Inherit: Same as input
  MATLAB Function : MATLAB Function  TreatAsAtomicUnit=on
  Mux2 : Mux
  Saturation1 : Saturate  UpperLimit=1  LowerLimit=-1
  Saturation2 : Saturate  UpperLimit=1  LowerLimit=-1
  Sum1 : Sum  InputSameDT=on  SaturateOnIntegerOverflow=on  OutDataTypeStr=Inherit: Same as first input
  Sum{5,8..10} (4 alike) : Sum  Inputs=-+  InputSameDT=on  SaturateOnIntegerOverflow=on  OutDataTypeStr=Inherit: Same as first input
  Sum11 : Sum  InputSameDT=on  SaturateOnIntegerOverflow=on  OutDataTypeStr=Inherit: Same as first input
  Sum2 : Sum  Inputs=+++  InputSameDT=on  SaturateOnIntegerOverflow=on  OutDataTypeStr=Inherit: Same as first input
  Switch : Switch  Criteria=u2 > Threshold
  Switch1 : Switch  Criteria=u2 > Threshold
  Switch2 : Switch  Criteria=u2 > Threshold
  Aileron : Outport
  Rudder : Outport  Port=2
  wires:
  Demux1/2 -> Sum11/2
  Roll/1 -> Sum10/2
  Sum5/1 -> Mux2/1
  Sum1/1 -> Saturation1/1
  sideslip_ref/1 -> Sum5/1
  Sum11/1 -> Saturation2/1
  sideslip/1 -> Sum5/2
  Saturation1/1 -> Aileron/1
  r/1 -> Sum9/2
  p/1 -> Sum8/2
  Sum9/1 -> Mux2/3
  p_ref/1 -> Sum8/1
  Aileron_trim/1 -> Sum1/1
  Roll_ref/1 -> Sum10/1
  Demux1/1 -> Sum1/2
  Rudder_trim/1 -> Sum11/1
  Saturation2/1 -> Rudder/1
  Sum10/1 -> Mux2/4
  r_ref/1 -> Sum9/1
  Sum8/1 -> Mux2/2
  th/1 -> MATLAB Function/1(th)
  Switch/1 -> LQR Gain1/1
  Switch1/1 -> LQR Gain2/1
  LQR Gain1/1 -> Sum2/1
  LQR Gain2/1 -> Sum2/2
  LQR Gain3/1 -> Sum2/3
  Switch2/1 -> LQR Gain3/1
  Sum2/1 -> Demux1/1
  Mux2/1 -> Switch2/1, Switch1/1, Switch/1
  Constant/1 -> Switch2/3, Switch1/3, Switch/3
  Demux/2 -> [B]
  MATLAB Function/1(y) -> Demux/1
  Demux/3 -> [C]
  Demux/1 -> [A]
  [A] -> Switch/2
  [B] -> Switch1/2
  [C] -> Switch2/2

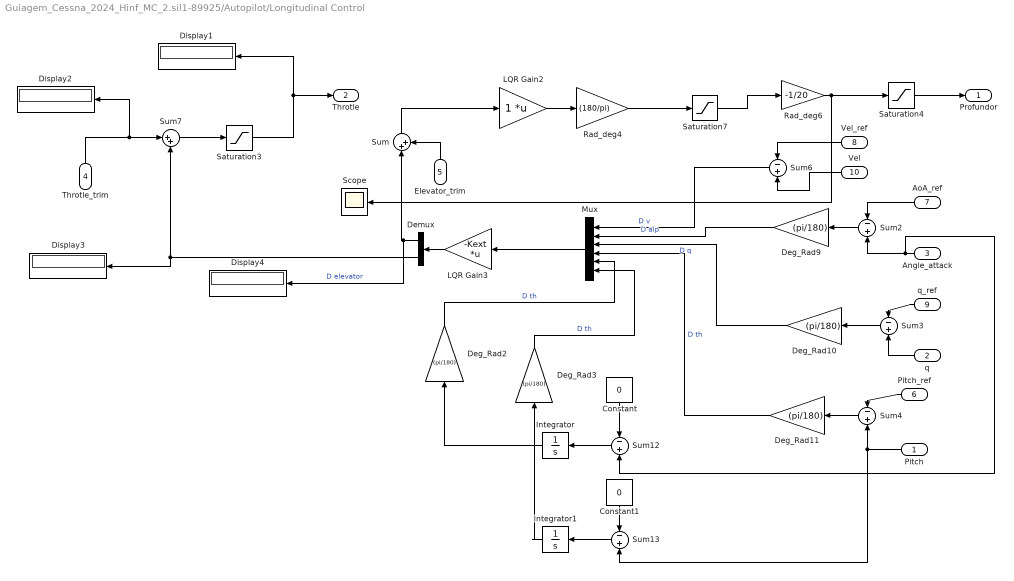
== system Guiagem_Cessna_2024_Hinf_MC_2.sil1-89925/Autopilot/Longitudinal Control ==
  Pitch : Inport
  q : Inport  Port=2
  Angle_attack : Inport  Port=3
  Throtle_trim : Inport  Port=4
  Elevator_trim : Inport  Port=5
  Pitch_ref : Inport  Port=6
  AoA_ref : Inport  Port=7
  Vel_ref : Inport  Port=8
  q_ref : Inport  Port=9
  Vel : Inport  Port=10
  Constant : Constant  Value=0
  Constant1 : Constant  Value=0
  Deg_Rad{2..3,9..11} (5 alike) : Gain  Gain=(pi/180)
  Demux : Demux  Outputs=2
  Display{1..4} (4 alike) : Display
  Integrator : Integrator
  Integrator1 : Integrator
  LQR Gain2 : Gain  Multiplication=Matrix(K*u)  SaturateOnIntegerOverflow=on  OutDataTypeStr=Inherit: Same as input  ParamDataTypeStr=Inherit: Same as input
  LQR Gain3 : Gain  Gain=-Kext  Multiplication=Matrix(K*u)  SaturateOnIntegerOverflow=on  OutDataTypeStr=Inherit: Same as input  ParamDataTypeStr=Inherit: Same as input
  Mux : Mux  Inputs=6
  Rad_deg4 : Gain  Gain=(180/pi)
  Rad_deg6 : Gain  Gain=-1/20
  Saturation3 : Saturate  UpperLimit=1  LowerLimit=0
  Saturation4 : Saturate
  Saturation7 : Saturate  UpperLimit=20  LowerLimit=-20
  Scope : Scope
  Sum : Sum  Inputs=|++
  Sum{2..4,6,12..13} (6 alike) : Sum  Inputs=-+  InputSameDT=on  SaturateOnIntegerOverflow=on  OutDataTypeStr=Inherit: Same as first input
  Sum7 : Sum  Inputs=|++
  Profundor : Outport
  Throtle : Outport  Port=2
  wires:
  Demux/1 -> Sum/1, Display4/1  "D elevator"
  Angle_attack/1 -> Sum2/2, Sum12/2
  Sum/1 -> LQR Gain2/1
  Pitch_ref/1 -> Sum4/1
  Integrator/1 -> Deg_Rad2/1
  Vel_ref/1 -> Sum6/1
  Sum12/1 -> Integrator/1
  Elevator_trim/1 -> Sum/2
  Saturation7/1 -> Rad_deg6/1
  Deg_Rad9/1 -> Mux/2  "D alp"
  Demux/2 -> Sum7/2, Display3/1
  Sum2/1 -> Deg_Rad9/1
  Saturation3/1 -> Display1/1, Throtle/1
  Throtle_trim/1 -> Display2/1, Sum7/1
  Deg_Rad2/1 -> Mux/5  "D th"
  Sum13/1 -> Integrator1/1
  LQR Gain2/1 -> Rad_deg4/1
  LQR Gain3/1 -> Demux/1
  Sum3/1 -> Deg_Rad10/1
  Sum7/1 -> Saturation3/1
  Constant1/1 -> Sum13/1
  Mux/1 -> LQR Gain3/1
  Constant/1 -> Sum12/1
  q/1 -> Sum3/2
  Deg_Rad3/1 -> Mux/6  "D th"
  Integrator1/1 -> Deg_Rad3/1
  Rad_deg6/1 -> Saturation4/1, Scope/1
  Pitch/1 -> Sum13/2, Sum4/2
  Sum4/1 -> Deg_Rad11/1
  Rad_deg4/1 -> Saturation7/1
  q_ref/1 -> Sum3/1
  Sum6/1 -> Mux/1  "D v"
  Saturation4/1 -> Profundor/1
  AoA_ref/1 -> Sum2/1
  Deg_Rad10/1 -> Mux/3  "D q"
  Deg_Rad11/1 -> Mux/4  "D th"
  Vel/1 -> Sum6/2

== system Guiagem_Cessna_2024_Hinf_MC_2.sil1-89925/Autopilot/Markov chain ==
  EN : Inport
  Constant : Constant
  Delay : Delay  DelayLength=1
  MATLAB Function : MATLAB Function  TreatAsAtomicUnit=on
  Scope1 : Scope
  Switch : Switch  Criteria=u2 > Threshold
  Uniform Random Number : UniformRandomNumber  Minimum=0
  th : Outport
  wires:
  MATLAB Function/1(next) -> Switch/1, Delay/1
  Delay/1 -> MATLAB Function/2(last)
  Uniform Random Number/1 -> MATLAB Function/1(rd)
  Switch/1 -> Scope1/1, th/1
  Constant/1 -> Switch/3
  EN/1 -> Switch/2

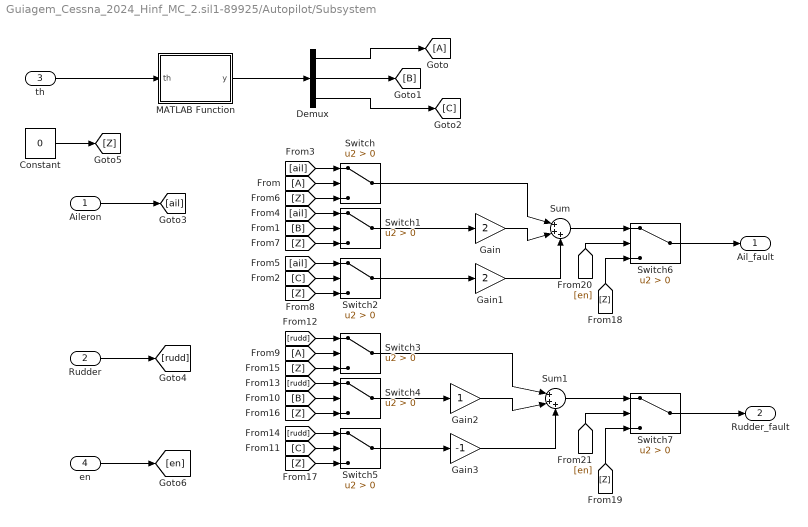
== system Guiagem_Cessna_2024_Hinf_MC_2.sil1-89925/Autopilot/Subsystem ==
  Aileron : Inport
  Rudder : Inport  Port=2
  th : Inport  Port=3
  en : Inport  Port=4
  Constant : Constant  Value=0
  Demux : Demux  Outputs=3
  Gain : Gain  Gain=2
  Gain1 : Gain  Gain=2
  Gain2 : Gain
  Gain3 : Gain  Gain=-1
  MATLAB Function : MATLAB Function  TreatAsAtomicUnit=on
  Sum : Sum  Inputs=|+++
  Sum1 : Sum  Inputs=|+++
  Switch{,1..7} (8 alike) : Switch  Criteria=u2 > Threshold
  Ail_fault : Outport
  Rudder_fault : Outport  Port=2
  wires:
  th/1 -> MATLAB Function/1(th)
  MATLAB Function/1(y) -> Demux/1
  Demux/1 -> [A]
  Demux/2 -> [B]
  Demux/3 -> [C]
  Aileron/1 -> [ail]
  Rudder/1 -> [rudd]
  [A] -> Switch/2
  [B] -> Switch1/2
  [C] -> Switch2/2
  [ail] -> Switch/1
  [ail] -> Switch1/1
  [ail] -> Switch2/1
  Constant/1 -> [Z]
  [Z] -> Switch/3
  [Z] -> Switch1/3
  [Z] -> Switch2/3
  Switch/1 -> Sum/1
  Switch1/1 -> Gain/1
  Switch2/1 -> Gain1/1
  Gain/1 -> Sum/2
  Gain1/1 -> Sum/3
  [Z] -> Switch3/3
  [rudd] -> Switch5/1
  [A] -> Switch3/2
  [rudd] -> Switch3/1
  [C] -> Switch5/2
  [Z] -> Switch5/3
  [B] -> Switch4/2
  [Z] -> Switch4/3
  [rudd] -> Switch4/1
  Switch4/1 -> Gain2/1
  Gain2/1 -> Sum1/2
  Switch3/1 -> Sum1/1
  Switch5/1 -> Gain3/1
  Gain3/1 -> Sum1/3
  Sum/1 -> Switch6/1
  Switch6/1 -> Ail_fault/1
  Sum1/1 -> Switch7/1
  Switch7/1 -> Rudder_fault/1
  [Z] -> Switch6/3
  [Z] -> Switch7/3
  en/1 -> [en]
  [en] -> Switch6/2
  [en] -> Switch7/2

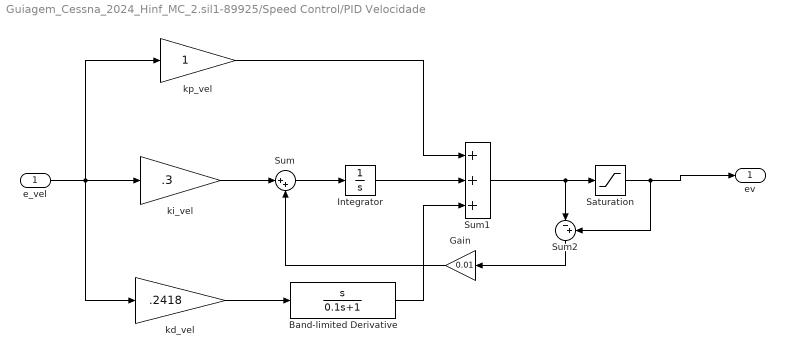
== system Guiagem_Cessna_2024_Hinf_MC_2.sil1-89925/Speed Control/PID Velocidade ==
  e_vel : Inport
  Band-limited Derivative : TransferFcn  Numerator=[1 0]  Denominator=[0.1 1]
  Gain : Gain  Gain=0.01
  Integrator : Integrator
  Saturation : Saturate  UpperLimit=1  LowerLimit=0
  Sum : Sum  Inputs=|++
  Sum1 : Sum  Inputs=+++  InputSameDT=on  SaturateOnIntegerOverflow=on  OutDataTypeStr=Inherit: Same as first input
  Sum2 : Sum  Inputs=|-+
  kd_vel : Gain  Gain=.2418  SaturateOnIntegerOverflow=on  OutDataTypeStr=Inherit: Same as input  ParamDataTypeStr=Inherit: Same as input
  ki_vel : Gain  Gain=.3  SaturateOnIntegerOverflow=on  OutDataTypeStr=Inherit: Same as input  ParamDataTypeStr=Inherit: Same as input
  kp_vel : Gain  SaturateOnIntegerOverflow=on  OutDataTypeStr=Inherit: Same as input  ParamDataTypeStr=Inherit: Same as input
  ev : Outport
  wires:
  kp_vel/1 -> Sum1/1
  Band-limited Derivative/1 -> Sum1/3
  e_vel/1 -> ki_vel/1, kp_vel/1, kd_vel/1
  kd_vel/1 -> Band-limited Derivative/1
  Integrator/1 -> Sum1/2
  Sum1/1 -> Sum2/1, Saturation/1
  ki_vel/1 -> Sum/1
  Sum/1 -> Integrator/1
  Gain/1 -> Sum/2
  Saturation/1 -> Sum2/2, ev/1
  Sum2/1 -> Gain/1

== matlab function Guiagem_Cessna_2024_Hinf_MC_2.sil1-89925/Autopilot/Markov chain/MATLAB Function ==
  data: rd input; next output; last input
function next = fcn(rd,last)

mu = [1 0 0 0 0 0];
P = [0.9500    0.0250         0    0.0250         0         0;
         0    0.9500    0.0250    0.0250         0         0;
         0         0    0.9500    0.0500         0         0;
    0.0350         0         0    0.9000    0.0500    0.0150;
    0.0700         0         0         0    0.9000    0.0300;
         0         0         0    0.1500         0    0.8500];
N= 6;
aux_next = 0;

if last == 0
    mu_aux = [0 cumsum(mu)];
    for i = 1:N
        if (mu_aux(i) <  rd)&&(rd <= mu_aux(i+1)) 
            aux_next = i;
        end
    end
else
    mu_aux = [0 cumsum(P(last,:))];
    for i = 1:N
        if (mu_aux(i) <  rd)&&(rd <= mu_aux(i+1)) 
            aux_next = i;
        end
    end
end
next = aux_next;

== matlab function Guiagem_Cessna_2024_Hinf_MC_2.sil1-89925/Autopilot/Command Center/MATLAB Function ==
  data: sel input; y output
function y = selector(sel)

N = 2;
y = zeros(N,1);

switch sel
    case 1 %% do nothing
        y(1) = 0;
    case 2 %% Markov on
        y(1) = 1;
    case 3 %% Initial On
        y(2) = 1;
    case 4 %% Markov & Initial On
        y = ones(2,1);    
    otherwise
        y = zeros(N,1);
end

== matlab function Guiagem_Cessna_2024_Hinf_MC_2.sil1-89925/Autopilot/Lateral Control/MATLAB Function ==
  data: th input; y output
function y = fault_select(th)

N = 3;
y = zeros(N,1);

switch th
    case 1
        y(1) = 1;
    case 2
        y(1) = 1;
    case 3
        y(1) = 1;
    case 4
        y(2) = 1;
    case 5
        y(2) = 1;
    case 6
        y(3) = 1;    
    otherwise
         y(1) = 1;
end

== matlab function Guiagem_Cessna_2024_Hinf_MC_2.sil1-89925/Autopilot/Du Bruit/MATLAB Function ==
  data: en input; w output; cnt input
function w = bruit(en,cnt)

w = 0;
Tf = 0.5;
CNT = Tf/0.01;
if en == 1 && cnt < CNT    
    w = 1;    
end

== matlab function Guiagem_Cessna_2024_Hinf_MC_2.sil1-89925/Autopilot/Subsystem/MATLAB Function ==
  data: th input; y output
function y = fault_select(th)

N = 3;
y = zeros(N,1);

switch th
    case 1
        y(1) = 1;
    case 2
        y(1) = 1;
    case 3
        y(1) = 1;
    case 4
        y(2) = 1;
    case 5
        y(2) = 1;
    case 6
        y(3) = 1;    
    otherwise
         y(1) = 1;
end
